simulink model "updated_target_driver_2026_withVariants_MPC_andwlqp2"  (R2024b)
settings: Solver=FixedStepDiscrete  StartTime=0.0  StopTime=running_time  FixedStep=dt_s  RelTol=1e-3
values from neighbouring files (symbols this model uses):
  A = gamma_2*gamma_3*Thrust_desired    [force2voltage.m]
  a2_lb = -0.25    [target_driver_setup_2022_Ctrl_V_2_4.m]    (also in target_driver_setup_2022_Ctrl_V_2_4_geometric.m; target_driver_setup_mpc_12msdelay.m; target_driver_setup_mpc_andWLQP.m)
  a2_openloop = -0    (= 0)    [target_driver_setup_2022_Ctrl_V_2_4.m]    (also in target_driver_setup_2022_Ctrl_V_2_4_geometric.m; target_driver_setup_mpc_12msdelay.m; target_driver_setup_mpc_andWLQP.m)
  a2_ub = 0.25    [target_driver_setup_2022_Ctrl_V_2_4.m]    (also in target_driver_setup_2022_Ctrl_V_2_4_geometric.m; target_driver_setup_mpc_12msdelay.m; target_driver_setup_mpc_andWLQP.m)
  att_s = 500    [target_driver_setup_2022_Ctrl_V_2_4.m]    (also in target_driver_setup_2022_Ctrl_V_2_4_geometric.m; target_driver_setup_mpc_12msdelay.m; target_driver_setup_mpc_andWLQP.m)
  c_vertical = 0.70e-3    (= 0.0007)    [target_driver_setup_mpc_andWLQP.m]
  closedloop_flag = 1    [target_driver_setup_2022_Ctrl_V_2_4.m]    (also in target_driver_setup_2022_Ctrl_V_2_4_geometric.m = 0; target_driver_setup_mpc_12msdelay.m = 0; target_driver_setup_mpc_andWLQP.m = 0)
  delay = delay-vicon_sample_cycle/2    [target_driver_setup_2022_Ctrl_V_2_4.m]    (also in target_driver_setup_2022_Ctrl_V_2_4_geometric.m; target_driver_setup_mpc_12msdelay.m; target_driver_setup_mpc_andWLQP.m)
  drv_amp = abs((vleft_p2p-vright_p2p))/2+min(vleft_p2p,vright_p2p)    [Wing_traj_to_Voltage.m]    (also in force2voltage.m; target_driver_setup_2022_Ctrl_V_2_4.m = 300; target_driver_setup_2022_Ctrl_V_2_4_geometric.m = 110; target_driver_setup_mpc_12msdelay.m = 150)
  drv_bias = max_drv_bias    (= 300)    [target_driver_setup_2022_Ctrl_V_2_4.m]    (also in target_driver_setup_2022_Ctrl_V_2_4_geometric.m = 200; target_driver_setup_mpc_12msdelay.m = 200; target_driver_setup_mpc_andWLQP.m = 200)
  drv_pitch_left = vleft_pitch    [Wing_traj_to_Voltage.m]    (also in force2voltage.m = 0; target_driver_setup_2022_Ctrl_V_2_4.m = 0; target_driver_setup_2022_Ctrl_V_2_4_geometric.m = 9.05; target_driver_setup_mpc_12msdelay.m = 9.05)
  drv_pitch_right = vright_pitch    [Wing_traj_to_Voltage.m]    (also in force2voltage.m = 0; target_driver_setup_2022_Ctrl_V_2_4.m = 0; target_driver_setup_2022_Ctrl_V_2_4_geometric.m = 9.05; target_driver_setup_mpc_12msdelay.m = 9.05)
  drv_roll = (vleft_p2p-vright_p2p)/4    [Wing_traj_to_Voltage.m]    (also in force2voltage.m; target_driver_setup_2022_Ctrl_V_2_4.m = 0; target_driver_setup_2022_Ctrl_V_2_4_geometric.m = -0.001; target_driver_setup_mpc_12msdelay.m = -0.001)
  dt_s = 1e-3    (= 0.001)    [target_driver_setup_2022_Ctrl_V_2_4.m]    (also in target_driver_setup_2022_Ctrl_V_2_4_geometric.m = 0.0002; target_driver_setup_mpc_12msdelay.m = 0.0002; target_driver_setup_mpc_andWLQP.m = 2.0e-4;1)
  f_fin = f    (= 180)    [target_driver_setup_2022_Ctrl_V_2_4.m]    (also in target_driver_setup_2022_Ctrl_V_2_4_geometric.m = 155; target_driver_setup_mpc_12msdelay.m = 155; target_driver_setup_mpc_andWLQP.m = 155)
  f_int = f    (= 180)    [target_driver_setup_2022_Ctrl_V_2_4.m]    (also in target_driver_setup_2022_Ctrl_V_2_4_geometric.m = 155; target_driver_setup_mpc_12msdelay.m = 155; target_driver_setup_mpc_andWLQP.m = 155)
  g = 9.8    [target_driver_setup_2022_Ctrl_V_2_4.m]    (also in target_driver_setup_2022_Ctrl_V_2_4_geometric.m; target_driver_setup_mpc_12msdelay.m; target_driver_setup_mpc_andWLQP.m = 9.81; test_full_attitude_mpc.m = 9.81)
  I_moment = eye(3)    [target_driver_exec_2022_Ctrl_V_2_4.m]    (also in target_driver_setup_2022_Ctrl_V_2_4.m; target_driver_setup_2022_Ctrl_V_2_4_geometric.m; target_driver_setup_mpc_12msdelay.m; target_driver_setup_mpc_andWLQP.m)
  k_tau_vec = [k_tau_roll;k_tau_pitch]    [target_driver_setup_2022_Ctrl_V_2_4_geometric.m]    (also in target_driver_setup_mpc_12msdelay.m; target_driver_setup_mpc_andWLQP.m)
  m = t <= t_zoom    [plot_roll_torque_cmd_vs_actual.m]    (also in plot_roll_torque_cmd_vs_actual_flightlog.m = t >= t0 & t <= t1; target_driver_setup_2022_Ctrl_V_2_4.m = 0.000124; target_driver_setup_2022_Ctrl_V_2_4_geometric.m = 8.5655e-05; target_driver_setup_mpc_12msdelay.m = 8.5655e-05)
  params_vec = [params_opt.delta_1, params_opt.delta_2, params_opt.delta_3,      params_opt.gamma_1, params_opt.gamma_2_1, params_opt.gamma_3,      params_opt.eta, params_opt.nu, params_opt.mu]'    [force2voltage_tuningSandbox.m]    (also in target_driver_setup_2022_Ctrl_V_2_4.m = [params_opt.delta_1, params_opt.delta_2, params_opt.delta_3,; target_driver_setup_2022_Ctrl_V_2_4_geometric.m = [params_opt.delta_1, params_opt.delta_2, params_opt.delta_3,; target_driver_setup_mpc_12msdelay.m = [params_opt.delta_1, params_opt.delta_2, params_opt.delta_3,; target_driver_setup_mpc_andWLQP.m = [params_opt.delta_1, params_opt.delta_2, params_opt.delta_3,)
  phase = 0    [target_driver_setup_2022_Ctrl_V_2_4.m]    (also in target_driver_setup_2022_Ctrl_V_2_4_geometric.m; target_driver_setup_mpc_12msdelay.m; target_driver_setup_mpc_andWLQP.m)
  popts_flattened = popts.popts    [target_driver_setup_mpc_andWLQP.m]
  roll_offset_angle = 0    [target_driver_setup_2022_Ctrl_V_2_4.m]    (also in target_driver_setup_2022_Ctrl_V_2_4_geometric.m; target_driver_setup_mpc_12msdelay.m; target_driver_setup_mpc_andWLQP.m)
  running_time = start_delay+total_T    (= 9)    [target_driver_setup_2022_Ctrl_V_2_4.m]    (also in target_driver_setup_2022_Ctrl_V_2_4_geometric.m = 10; target_driver_setup_mpc_12msdelay.m = 0.5; target_driver_setup_mpc_andWLQP.m = 10)
  running_time_control = start_delay_control+total_T+0.0    (= 7.1)    [target_driver_setup_2022_Ctrl_V_2_4.m]    (also in target_driver_setup_2022_Ctrl_V_2_4_geometric.m = 10; target_driver_setup_mpc_12msdelay.m = 0.5; target_driver_setup_mpc_andWLQP.m = 10)
  sampling_f = 10000    [target_driver_setup_2022_Ctrl_V_2_4.m]    (also in target_driver_setup_2022_Ctrl_V_2_4_geometric.m = 5000; target_driver_setup_mpc_12msdelay.m = 5000; target_driver_setup_mpc_andWLQP.m = 1/dt_s)
  start_delay = 2.0    (= 2)    [target_driver_setup_2022_Ctrl_V_2_4.m]    (also in target_driver_setup_2022_Ctrl_V_2_4_geometric.m = 0; target_driver_setup_mpc_12msdelay.m = 0; target_driver_setup_mpc_andWLQP.m = 0)
  start_delay_control = start_delay + ramp_delay    (= 0.1)    [target_driver_setup_2022_Ctrl_V_2_4.m]    (also in target_driver_setup_2022_Ctrl_V_2_4_geometric.m = 0; target_driver_setup_mpc_12msdelay.m = 0; target_driver_setup_mpc_andWLQP.m = 0)
  T = 1    [target_driver_setup_2022_Ctrl_V_2_4.m]    (also in target_driver_setup_2022_Ctrl_V_2_4_geometric.m = 10; target_driver_setup_mpc_12msdelay.m = 0.5; target_driver_setup_mpc_andWLQP.m = 10; test_full_attitude_mpc.m = T0 + nu(1))
  weights_vec = [ws; wds; wpr_xy;wpr_z; wpf; wvr_xy; wvr_z ... (first row only)    [target_driver_setup_2022_Ctrl_V_2_4_geometric.m]    (also in target_driver_setup_mpc_12msdelay.m; target_driver_setup_mpc_andWLQP.m)
undefined symbols (not defined in the file or in its folder): Com1, ctrl_Ts, DiscIntNeverNeededParam, dspblkCoreblockFVToolHelper, gcbh, left_mapping, left_mapping_F_to_Phi, lp_den, lp_num, none, right_mapping, right_mapping_F_to_Phi
libraries: simulink x17, xpcseriallib x2, cstblocks x1, xpcnilib x1, xpcutilitieslib x1
(part 3 of 4)

== system updated_target_driver_2026_withVariants_MPC_andwlqp2/Variant Subsystem/Simulation/signal generator a3/Drive_Signal/AveragedOffset_filtered ==
  note: To avoid having signal "jump",
      | we want SMOOTH transitions
      | in frequency (i.e., a weighted sum
      | of current freq and freq some delta t ago)
  note: time constant 0.02sec
      | for 10kHz samping
  In1 : Inport
  Discrete Transfer Fcn : DiscreteTransferFcn  LoadFcn=dspblkCoreblockFVToolHelper(gcbh,'load');  Numerator=[0.05]  Denominator=[1 -.95]
      settings: CopyFcn=dspblkCoreblockFVToolHelper(gcbh,'copy');  DeleteFcn=dspblkCoreblockFVToolHelper(gcbh,'close');  ModelCloseFcn=dspblkCoreblockFVToolHelper(gcbh,'close');  PreSaveFcn=dspblkCoreblockFVToolHelper(gcbh,'presave');  PostSaveFcn=dspblkCoreblockFVToolHelper(gcbh,'postsave');  CloseFcn=dspblkCoreblockFVToolHelper(gcbh,'close');
  Discrete Transfer Fcn2 : DiscreteTransferFcn  LoadFcn=dspblkCoreblockFVToolHelper(gcbh,'load');  Numerator=[0.37152]  Denominator=[1 -.62848]
      settings: CopyFcn=dspblkCoreblockFVToolHelper(gcbh,'copy');  DeleteFcn=dspblkCoreblockFVToolHelper(gcbh,'close');  ModelCloseFcn=dspblkCoreblockFVToolHelper(gcbh,'close');  PreSaveFcn=dspblkCoreblockFVToolHelper(gcbh,'presave');  PostSaveFcn=dspblkCoreblockFVToolHelper(gcbh,'postsave');  CloseFcn=dspblkCoreblockFVToolHelper(gcbh,'close');
  Out1 : Outport
  wires:
  In1/1 -> Discrete Transfer Fcn2/1
  Discrete Transfer Fcn2/1 -> Out1/1

== system updated_target_driver_2026_withVariants_MPC_andwlqp2/Variant Subsystem/Simulation/signal generator a3/Drive_Signal/FlattenedSine1 ==
  freq : Inport
  phase : Inport  Port=2
  a2 : Inport  Port=3
  0.1 : Gain  Gain=0.1
  1.1 : Gain  Gain=1.1
  2f : Gain  Gain=2
  2pi : Gain  Gain=2*pi
  3f : Gain  Gain=3
  Add : Sum  Inputs=+++
  Add1 : Sum
  Amplitude Correction : Subsystem  Commented=on
  AveragedAmp_filtered : Subsystem
  Product : Product
  first harmonic : Trigonometry  OutputSignalType=real
  integrate(omega*t) : DiscreteIntegrator  SampleTime=-1  ICPrevOutput=DiscIntNeverNeededParam  ICPrevScaledInput=DiscIntNeverNeededParam
  second harmonic : Trigonometry  OutputSignalType=real
  third harmonic : Trigonometry  OutputSignalType=real
  split cycle signal : Outport
  wires:
  freq/1 -> 2pi/1
  2pi/1 -> integrate(omega*t)/1
  3f/1 -> third harmonic/1
  first harmonic/1 -> 1.1/1
  third harmonic/1 -> 0.1/1
  1.1/1 -> Add/1
  Add1/1 -> first harmonic/1, 2f/1, 3f/1
  integrate(omega*t)/1 -> Add1/1
  phase/1 -> Add1/2
  2f/1 -> second harmonic/1
  0.1/1 -> Add/2
  Product/1 -> Add/3
  second harmonic/1 -> Product/1
  Add/1 -> split cycle signal/1
  a2/1 -> AveragedAmp_filtered/1(In1)
  AveragedAmp_filtered/1(Out1) -> Product/2

== system updated_target_driver_2026_withVariants_MPC_andwlqp2/Variant Subsystem/Simulation/signal generator a3/Drive_Signal/FlattenedSine_phase ==
  f : Inport
  phase : Inport  Port=2
  0.1 : Gain  Gain=0.1
  1.1 : Gain  Gain=1.1
  2pi : Gain  Gain=2*pi
  3f : Gain  Gain=3
  Add : Sum
  Sum : Sum  Inputs=|++
  first harmonic : Trigonometry  OutputSignalType=real
  integrate(omega*t) : DiscreteIntegrator  SampleTime=-1  ICPrevOutput=DiscIntNeverNeededParam  ICPrevScaledInput=DiscIntNeverNeededParam
  pi/180 : Gain  Gain=pi/180
  third harmonic : Trigonometry  OutputSignalType=real
  split cycle signal : Outport
  wires:
  f/1 -> 2pi/1
  2pi/1 -> integrate(omega*t)/1
  3f/1 -> third harmonic/1
  first harmonic/1 -> 1.1/1
  third harmonic/1 -> 0.1/1
  1.1/1 -> Add/1
  0.1/1 -> Add/2
  Add/1 -> split cycle signal/1
  Sum/1 -> first harmonic/1, 3f/1
  pi/180/1 -> Sum/2
  integrate(omega*t)/1 -> Sum/1
  phase/1 -> pi/180/1

== system updated_target_driver_2026_withVariants_MPC_andwlqp2/Variant Subsystem/Simulation/signal generator a3/Drive_Signal/SignalForRamp_binary ==
  note: Should output 1 or -1,
      | so signal ramps UP to 1
      | or DOWN to 0.
  In1 : Inport
  Add : Sum  Inputs=+-
  Compare To Zero : simulink/Logic and Bit Operations/Compare To Zero  relop=>  OutDataTypeStr=uint8  ZeroCross=off
  Constant : Constant
  Data Type Conversion : DataTypeConversion  OutDataTypeStr=double  SaturateOnIntegerOverflow=off  RndMeth=Floor
  Gain : Gain  Gain=2
  Out1 : Outport
  wires:
  In1/1 -> Compare To Zero/1
  Compare To Zero/1 -> Data Type Conversion/1
  Gain/1 -> Add/1
  Constant/1 -> Add/2
  Add/1 -> Out1/1
  Data Type Conversion/1 -> Gain/1

== system updated_target_driver_2026_withVariants_MPC_andwlqp2/Variant Subsystem/Simulation/signal generator a3/Drive_Signal/SignalForSin_binary ==
  note: We want this to stay "high" for 1
      | second after the actual "enable"
      | is turned off...
  In1 : Inport
  Compare To Zero : simulink/Logic and Bit Operations/Compare To Zero  relop=>  OutDataTypeStr=uint8  ZeroCross=off
  Data Type Conversion : DataTypeConversion  OutDataTypeStr=double  SaturateOnIntegerOverflow=off  RndMeth=Floor
  Out1 : Outport
  wires:
  In1/1 -> Compare To Zero/1
  Compare To Zero/1 -> Data Type Conversion/1
  Data Type Conversion/1 -> Out1/1

== system updated_target_driver_2026_withVariants_MPC_andwlqp2/Variant Subsystem/Simulation/signal generator a3/Drive_Signal/Sinewave ==
  In2 : Inport
  2pi : Gain  Gain=2*pi
  first harmonic : Trigonometry  OutputSignalType=real
  integrate(omega*t) : DiscreteIntegrator  SampleTime=-1  ICPrevOutput=DiscIntNeverNeededParam  ICPrevScaledInput=DiscIntNeverNeededParam
  split cycle signal : Outport
  wires:
  In2/1 -> 2pi/1
  2pi/1 -> integrate(omega*t)/1
  integrate(omega*t)/1 -> first harmonic/1
  first harmonic/1 -> split cycle signal/1

== system updated_target_driver_2026_withVariants_MPC_andwlqp2/Variant Subsystem/Simulation/signal generator a3/Drive_Signal1/AveragedAmp_filtered ==
  note: To avoid having signal "jump",
      | we want SMOOTH transitions
      | in frequency (i.e., a weighted sum
      | of current freq and freq some delta t ago)
  note: time constant 0.002sec
      | for 10kHz samping
  In1 : Inport
  Discrete Transfer Fcn1 : DiscreteTransferFcn  LoadFcn=dspblkCoreblockFVToolHelper(gcbh,'load');  Numerator=[0.05]  Denominator=[1 -.95]
      settings: CopyFcn=dspblkCoreblockFVToolHelper(gcbh,'copy');  DeleteFcn=dspblkCoreblockFVToolHelper(gcbh,'close');  ModelCloseFcn=dspblkCoreblockFVToolHelper(gcbh,'close');  PreSaveFcn=dspblkCoreblockFVToolHelper(gcbh,'presave');  PostSaveFcn=dspblkCoreblockFVToolHelper(gcbh,'postsave');  CloseFcn=dspblkCoreblockFVToolHelper(gcbh,'close');
  Discrete Transfer Fcn2 : DiscreteTransferFcn  LoadFcn=dspblkCoreblockFVToolHelper(gcbh,'load');  Numerator=[0.37152]  Denominator=[1 -.62848]
      settings: CopyFcn=dspblkCoreblockFVToolHelper(gcbh,'copy');  DeleteFcn=dspblkCoreblockFVToolHelper(gcbh,'close');  ModelCloseFcn=dspblkCoreblockFVToolHelper(gcbh,'close');  PreSaveFcn=dspblkCoreblockFVToolHelper(gcbh,'presave');  PostSaveFcn=dspblkCoreblockFVToolHelper(gcbh,'postsave');  CloseFcn=dspblkCoreblockFVToolHelper(gcbh,'close');
  Out1 : Outport
  wires:
  In1/1 -> Discrete Transfer Fcn2/1
  Discrete Transfer Fcn2/1 -> Out1/1

== system updated_target_driver_2026_withVariants_MPC_andwlqp2/Variant Subsystem/Simulation/signal generator a3/Drive_Signal1/AveragedOffset_filtered ==
  note: To avoid having signal "jump",
      | we want SMOOTH transitions
      | in frequency (i.e., a weighted sum
      | of current freq and freq some delta t ago)
  note: c
  note: time constant 0.02sec
      | for 10kHz samping
  In1 : Inport
  Discrete Transfer Fcn1 : DiscreteTransferFcn  LoadFcn=dspblkCoreblockFVToolHelper(gcbh,'load');  Numerator=[0.05]  Denominator=[1 -.95]
      settings: CopyFcn=dspblkCoreblockFVToolHelper(gcbh,'copy');  DeleteFcn=dspblkCoreblockFVToolHelper(gcbh,'close');  ModelCloseFcn=dspblkCoreblockFVToolHelper(gcbh,'close');  PreSaveFcn=dspblkCoreblockFVToolHelper(gcbh,'presave');  PostSaveFcn=dspblkCoreblockFVToolHelper(gcbh,'postsave');  CloseFcn=dspblkCoreblockFVToolHelper(gcbh,'close');
  Discrete Transfer Fcn2 : DiscreteTransferFcn  LoadFcn=dspblkCoreblockFVToolHelper(gcbh,'load');  Numerator=[0.37152]  Denominator=[1 -.62848]
      settings: CopyFcn=dspblkCoreblockFVToolHelper(gcbh,'copy');  DeleteFcn=dspblkCoreblockFVToolHelper(gcbh,'close');  ModelCloseFcn=dspblkCoreblockFVToolHelper(gcbh,'close');  PreSaveFcn=dspblkCoreblockFVToolHelper(gcbh,'presave');  PostSaveFcn=dspblkCoreblockFVToolHelper(gcbh,'postsave');  CloseFcn=dspblkCoreblockFVToolHelper(gcbh,'close');
  Out1 : Outport
  wires:
  In1/1 -> Discrete Transfer Fcn2/1
  Discrete Transfer Fcn2/1 -> Out1/1

== system updated_target_driver_2026_withVariants_MPC_andwlqp2/Variant Subsystem/Simulation/signal generator a3/Drive_Signal1/FlattenedSine1 ==
  freq : Inport
  a2 : Inport  Port=2
  0.1 : Gain  Gain=0.1
  1.1 : Gain  Gain=1.1
  2f : Gain  Gain=2
  2pi : Gain  Gain=2*pi
  3f : Gain  Gain=3
  Add : Sum  Inputs=+++
  Amplitude Correction : Subsystem  Commented=on
  AveragedAmp_filtered : Subsystem
  Product : Product
  first harmonic : Trigonometry  OutputSignalType=real
  flip : Gain  Gain=-1
  integrate(omega*t) : DiscreteIntegrator  SampleTime=-1  ICPrevOutput=DiscIntNeverNeededParam  ICPrevScaledInput=DiscIntNeverNeededParam
  second harmonic : Trigonometry  OutputSignalType=real
  third harmonic : Trigonometry  OutputSignalType=real
  split cycle signal : Outport
  wires:
  freq/1 -> 2pi/1
  2pi/1 -> integrate(omega*t)/1
  3f/1 -> third harmonic/1
  first harmonic/1 -> 1.1/1
  third harmonic/1 -> 0.1/1
  1.1/1 -> Add/1
  integrate(omega*t)/1 -> first harmonic/1, 2f/1, 3f/1
  2f/1 -> second harmonic/1
  0.1/1 -> Add/2
  Product/1 -> Add/3
  second harmonic/1 -> Product/1
  flip/1 -> Product/2
  Add/1 -> split cycle signal/1
  a2/1 -> AveragedAmp_filtered/1(In1)
  AveragedAmp_filtered/1(Out1) -> flip/1

== system updated_target_driver_2026_withVariants_MPC_andwlqp2/Variant Subsystem/Simulation/signal generator a3/Drive_Signal1/SignalForRamp_binary ==
  note: Should output 1 or -1,
      | so signal ramps UP to 1
      | or DOWN to 0.
  In1 : Inport
  Add : Sum  Inputs=+-
  Compare To Zero : simulink/Logic and Bit Operations/Compare To Zero  relop=>  OutDataTypeStr=uint8  ZeroCross=off
  Constant : Constant
  Data Type Conversion : DataTypeConversion  OutDataTypeStr=double  SaturateOnIntegerOverflow=off  RndMeth=Floor
  Gain : Gain  Gain=2
  Out1 : Outport
  wires:
  In1/1 -> Compare To Zero/1
  Compare To Zero/1 -> Data Type Conversion/1
  Gain/1 -> Add/1
  Constant/1 -> Add/2
  Add/1 -> Out1/1
  Data Type Conversion/1 -> Gain/1

== system updated_target_driver_2026_withVariants_MPC_andwlqp2/Variant Subsystem/Simulation/signal generator a3/Drive_Signal1/SignalForSin_binary ==
  note: We want this to stay "high" for 1
      | second after the actual "enable"
      | is turned off...
  In1 : Inport
  Compare To Zero : simulink/Logic and Bit Operations/Compare To Zero  relop=>  OutDataTypeStr=uint8  ZeroCross=off
  Data Type Conversion : DataTypeConversion  OutDataTypeStr=double  SaturateOnIntegerOverflow=off  RndMeth=Floor
  Out1 : Outport
  wires:
  In1/1 -> Compare To Zero/1
  Compare To Zero/1 -> Data Type Conversion/1
  Data Type Conversion/1 -> Out1/1

== system updated_target_driver_2026_withVariants_MPC_andwlqp2/Variant Subsystem/Simulation/signal generator a3/Drive_Signal1/Sine Wave ==
  In2 : Inport
  2pi : Gain  Gain=2*pi
  first harmonic : Trigonometry  OutputSignalType=real
  integrate(omega*t) : DiscreteIntegrator  SampleTime=-1  ICPrevOutput=DiscIntNeverNeededParam  ICPrevScaledInput=DiscIntNeverNeededParam
  split cycle signal : Outport
  wires:
  In2/1 -> 2pi/1
  2pi/1 -> integrate(omega*t)/1
  integrate(omega*t)/1 -> first harmonic/1
  first harmonic/1 -> split cycle signal/1

== system updated_target_driver_2026_withVariants_MPC_andwlqp2/Variant Subsystem/Experimental/signal generator a3/Drive_Signal/FlattenedSine1/Amplitude Correction ==
  y : Inport
  a2 : Inport  Port=2
  Abs : Abs  SaturateOnIntegerOverflow=off
  Constant : Constant  Value=1.2
  Constant1 : Constant  Value=1.1
  Divide : Product  Inputs=*/
  Product1 : Product
  Sqrt : Sqrt
  Subtract : Sum  Inputs=+-
  y_new : Outport
  wires:
  Constant/1 -> Subtract/1
  Subtract/1 -> Sqrt/1
  Abs/1 -> Subtract/2
  a2/1 -> Abs/1
  y/1 -> Product1/1
  Product1/1 -> y_new/1
  Divide/1 -> Product1/2
  Constant1/1 -> Divide/2
  Sqrt/1 -> Divide/1

== system updated_target_driver_2026_withVariants_MPC_andwlqp2/Variant Subsystem/Experimental/signal generator a3/Drive_Signal/FlattenedSine1/AveragedAmp_filtered ==
  note: To avoid having signal "jump",
      | we want SMOOTH transitions
      | in frequency (i.e., a weighted sum
      | of current freq and freq some delta t ago)
  note: time constant 0.002sec
      | for 10kHz samping
  In1 : Inport
  Discrete Transfer Fcn : DiscreteTransferFcn  Numerator=[0.05]  Denominator=[1 -.95]
  Out1 : Outport
  wires:
  In1/1 -> Discrete Transfer Fcn/1
  Discrete Transfer Fcn/1 -> Out1/1

== system updated_target_driver_2026_withVariants_MPC_andwlqp2/Variant Subsystem/Experimental/signal generator a3/Drive_Signal1/FlattenedSine1/Amplitude Correction ==
  y : Inport
  a2 : Inport  Port=2
  Abs : Abs  SaturateOnIntegerOverflow=off
  Constant : Constant  Value=1.2
  Constant1 : Constant  Value=1.1
  Divide : Product  Inputs=*/
  Product1 : Product
  Sqrt : Sqrt
  Subtract : Sum  Inputs=+-
  y_new : Outport
  wires:
  Constant/1 -> Subtract/1
  Subtract/1 -> Sqrt/1
  Abs/1 -> Subtract/2
  a2/1 -> Abs/1
  y/1 -> Product1/1
  Product1/1 -> y_new/1
  Divide/1 -> Product1/2
  Constant1/1 -> Divide/2
  Sqrt/1 -> Divide/1

== system updated_target_driver_2026_withVariants_MPC_andwlqp2/Variant Subsystem/Experimental/signal generator a3/Drive_Signal1/FlattenedSine1/AveragedAmp_filtered ==
  note: To avoid having signal "jump",
      | we want SMOOTH transitions
      | in frequency (i.e., a weighted sum
      | of current freq and freq some delta t ago)
  note: time constant 0.002sec
      | for 10kHz samping
  In1 : Inport
  Discrete Transfer Fcn : DiscreteTransferFcn  Numerator=[0.05]  Denominator=[1 -.95]
  Out1 : Outport
  wires:
  In1/1 -> Discrete Transfer Fcn/1
  Discrete Transfer Fcn/1 -> Out1/1

== system updated_target_driver_2026_withVariants_MPC_andwlqp2/Variant Subsystem/Simulation/signal generator a3/Drive_Signal/FlattenedSine1/Amplitude Correction ==
  y : Inport
  a2 : Inport  Port=2
  Abs : Abs  SaturateOnIntegerOverflow=off
  Constant : Constant  Value=1.2
  Constant1 : Constant  Value=1.1
  Divide : Product  Inputs=*/
  Product1 : Product
  Sqrt : Sqrt
  Subtract : Sum  Inputs=+-
  y_new : Outport
  wires:
  Constant/1 -> Subtract/1
  Subtract/1 -> Sqrt/1
  Abs/1 -> Subtract/2
  a2/1 -> Abs/1
  y/1 -> Product1/1
  Product1/1 -> y_new/1
  Divide/1 -> Product1/2
  Constant1/1 -> Divide/2
  Sqrt/1 -> Divide/1

== system updated_target_driver_2026_withVariants_MPC_andwlqp2/Variant Subsystem/Simulation/signal generator a3/Drive_Signal/FlattenedSine1/AveragedAmp_filtered ==
  note: To avoid having signal "jump",
      | we want SMOOTH transitions
      | in frequency (i.e., a weighted sum
      | of current freq and freq some delta t ago)
  note: time constant 0.002sec
      | for 10kHz samping
  In1 : Inport
  Discrete Transfer Fcn : DiscreteTransferFcn  Numerator=[0.05]  Denominator=[1 -.95]
  Out1 : Outport
  wires:
  In1/1 -> Discrete Transfer Fcn/1
  Discrete Transfer Fcn/1 -> Out1/1

== system updated_target_driver_2026_withVariants_MPC_andwlqp2/Variant Subsystem/Simulation/signal generator a3/Drive_Signal1/FlattenedSine1/Amplitude Correction ==
  y : Inport
  a2 : Inport  Port=2
  Abs : Abs  SaturateOnIntegerOverflow=off
  Constant : Constant  Value=1.2
  Constant1 : Constant  Value=1.1
  Divide : Product  Inputs=*/
  Product1 : Product
  Sqrt : Sqrt
  Subtract : Sum  Inputs=+-
  y_new : Outport
  wires:
  Constant/1 -> Subtract/1
  Subtract/1 -> Sqrt/1
  Abs/1 -> Subtract/2
  a2/1 -> Abs/1
  y/1 -> Product1/1
  Product1/1 -> y_new/1
  Divide/1 -> Product1/2
  Constant1/1 -> Divide/2
  Sqrt/1 -> Divide/1

== system updated_target_driver_2026_withVariants_MPC_andwlqp2/Variant Subsystem/Simulation/signal generator a3/Drive_Signal1/FlattenedSine1/AveragedAmp_filtered ==
  note: To avoid having signal "jump",
      | we want SMOOTH transitions
      | in frequency (i.e., a weighted sum
      | of current freq and freq some delta t ago)
  note: time constant 0.002sec
      | for 10kHz samping
  In1 : Inport
  Discrete Transfer Fcn : DiscreteTransferFcn  Numerator=[0.05]  Denominator=[1 -.95]
  Out1 : Outport
  wires:
  In1/1 -> Discrete Transfer Fcn/1
  Discrete Transfer Fcn/1 -> Out1/1

== matlab function updated_target_driver_2026_withVariants_MPC_andwlqp2/Variant Subsystem/Simulation/Drake 2 Controller Axes1 ==
  data: x_drake input; x output; y_drake input; z_drake input; y output; z output
function [x,y,z] = fcn(x_drake,y_drake,z_drake)

    [x,y,z] = drake2controllerposition(x_drake,y_drake,z_drake); 

end

== matlab function updated_target_driver_2026_withVariants_MPC_andwlqp2/MATLAB Function1 ==
  data: R_cur input size=9; pdotdes output size=6; omega input size=3; p_cur input size=3; v_cur input size=3; pdes input size=3; dpdes input size=3; sdes_in input size=3; I_moment_vec input size=3; m input size=1; g input size=1; cntrl_enable input size=1; weights_vec input size=14; k_tau input size=2; ctrl_Ts input size=1; h0_wl output size=6; accdes output size=6; thrust_desired output size=1; roll_torque_desired output size=1; pitch_torque_desired output size=1; yaw_torque_desired output size=1; a_ref input; yaw_ref input
function [pdotdes, h0_wl, accdes, thrust_desired, roll_torque_desired, ...
    pitch_torque_desired, yaw_torque_desired] = fcn( ...
    R_cur, omega, p_cur, v_cur, pdes, dpdes, sdes_in, ...
    I_moment_vec, m, g, cntrl_enable, weights_vec, k_tau, ctrl_Ts, a_ref, yaw_ref) 

%#codegen
    [pdotdes, h0_wl, accdes, thrust_desired, roll_torque_desired, ...
    pitch_torque_desired, yaw_torque_desired] = upright_template_mpc_wl( ...
    R_cur, omega, p_cur, v_cur, pdes, dpdes, sdes_in, ...
    I_moment_vec, m, g, cntrl_enable, weights_vec, k_tau, ctrl_Ts, a_ref, yaw_ref); 

end

== matlab function updated_target_driver_2026_withVariants_MPC_andwlqp2/wlqp2driver ==
  data: u input size=4; drv_amp output size=1; drv_pitch_left output size=1; drv_pitch_right output size=1; drv_roll output size=1; a2 output size=1; signs input size=3; drv_bias output size=1; vleft output size=1; vright output size=1
function [drv_amp, drv_pitch_left, drv_pitch_right, drv_roll, a2, ...
    drv_bias, vleft, vright] = fcn(u, signs)
    [drv_amp, drv_pitch_left, drv_pitch_right, drv_roll, a2, ...
    drv_bias, vleft, vright] = wlqp2driver(u, signs);
end

== matlab function updated_target_driver_2026_withVariants_MPC_andwlqp2/Force to voltage/Control Mode/Force_to_Voltage1/Desired_Force_to_Voltage ==
  data: Thrust_desired input; drv_amp output; Roll_torque_desired input; Pitch_torque_desired input; Yaw_torque_desired input; drv_roll output; drv_pitch_left output; drv_pitch_right output; a2_coeff output; params_vec input
function [drv_amp, drv_roll, drv_pitch_left, drv_pitch_right, a2_coeff] =    fcn(Thrust_desired, Roll_torque_desired, Pitch_torque_desired, Yaw_torque_desired, params_vec)

% 
% Thrust_desired = 0.7e-3;% N
% Roll_torque_desired = 20e-6; %mN mm 
% Pitch_torque_desired = 0;% N  
% Yaw_torque_desired = 0;  
[drv_amp, drv_roll, drv_pitch_left, drv_pitch_right, a2_coeff] = force2voltage( ...
    Thrust_desired, Roll_torque_desired, Pitch_torque_desired, ...
    Yaw_torque_desired, params_vec);
% % global params_opt
% 
% delta_1 = params_vec(1);
% delta_2 = params_vec(2);
% delta_3 = params_vec(3);
% gamma_1 = params_vec(4);
% gamma_2 = params_vec(5);
% gamma_3 = params_vec(6);
% eta = params_vec(7);
% nu = params_vec(8);
% mu = params_vec(9);
% 
% 
% % Initializing for averaging filter at the end to prevent InF
% if Thrust_desired==0    
%     u4 = 0;
% else
%     u4 = Pitch_torque_desired/(Thrust_desired*delta_3*gamma_2)-nu;
% end
% 
% 
% % u3 calculation when tau approaches to zero
% if abs(Yaw_torque_desired)<1e-12
% 
%    u3 = -mu;
% else
%     % Bounds for the mapping to produce real solution
%     lb =(Thrust_desired/2)*(gamma_2*gamma_3*delta_2*mu/delta_1-sqrt((gamma_2*gamma_3*delta_2*Thrust_desired*mu/delta_1)^2+gamma_2*gamma_3));
%     ub =(Thrust_desired/2)*(gamma_2*gamma_3*delta_2*mu/delta_1+sqrt((gamma_2*gamma_3*delta_2*Thrust_desired*mu/delta_1)^2+gamma_2*gamma_3));
% 
%     if Yaw_torque_desired>=ub
%        Yaw_torque_desired = ub;
%     elseif Yaw_torque_desired<=lb
%        Yaw_torque_desired = lb; 
%     end
% 
%     % u3 calculation when tau approaches zero
%     if abs(Yaw_torque_desired) < 1e-12
%         u3 = -mu;
%     else
%         A = gamma_2*gamma_3*Thrust_desired;
%         B = gamma_2*gamma_3*delta_2*Thrust_desired*mu/delta_1;
% 
%         disc = A^2 - 4*Yaw_torque_desired*(Yaw_torque_desired - B);
% 
%     % Numerical / feasibility guard
%     if disc < 0
%         disc = 0;
%     end
% 
%     u3 = delta_1*(A - sqrt(disc))/(2*delta_2*Yaw_torque_desired);
%     end
% end
% 
% D = delta_1^2+delta_2^2*u3^2;
% % gamma_2*Thrust_desired+Roll_torque_desired 
% u1 = (gamma_2*Thrust_desired+Roll_torque_desired)/(2*gamma_1*gamma_2*D*eta);
% u2 = (gamma_2*Thrust_desired-Roll_torque_desired)/(2*gamma_1*gamma_2*D);
% 
% u1 = max(u1, 0); 
% u2 = max(u2, 0); % Guard against negative voltage
% vleft_p2p = sqrt(u1)*2; 
% vright_p2p = sqrt(u2)*2;
% vleft_pitch = u4;
% vright_pitch = u4;
% 
% 
% drv_amp = abs((vleft_p2p-vright_p2p))/2+min(vleft_p2p,vright_p2p); % p2p
% drv_roll = (vleft_p2p-vright_p2p)/4; % Amplitude
% drv_pitch_left = vleft_pitch;
% drv_pitch_right = vright_pitch;
% a2_coeff = u3;
% 
end

== matlab function updated_target_driver_2026_withVariants_MPC_andwlqp2/MATLAB Function2 ==
  data: Rot_corrected_vec input; wrenchBias output; v_filtered_W input; c_vertical_N_per_mps input
function wrenchBias = wlqp_vertical_wrench_bias(Rot_corrected_vec, v_filtered_W, c_vertical_N_per_mps)
%#codegen
    wrenchBias = wlqp_vertical_wrench_bias( ...
    Rot_corrected_vec, v_filtered_W, c_vertical_N_per_mps); 
end 

% y = u;

== matlab function updated_target_driver_2026_withVariants_MPC_andwlqp2/Force to voltage/Control Mode/Force_to_Voltage1/Force to Trajectory  ==
  data: Thrust_desired input; Phi_left_p2p_desired output; Roll_torque_desired input; Pitch_torque_desired input; left_mapping_F_to_Phi input; right_mapping_F_to_Phi input; A input; Phi_right_p2p_desired output; Phi_pitch_desired output
function [Phi_left_p2p_desired, Phi_right_p2p_desired, Phi_pitch_desired] = fcn(Thrust_desired, Roll_torque_desired, Pitch_torque_desired, left_mapping_F_to_Phi, right_mapping_F_to_Phi, A)

delta_opt_L = left_mapping_F_to_Phi(1);
gamma_opt_L = left_mapping_F_to_Phi(2);
phi_opt_L = left_mapping_F_to_Phi(3);
phi_opt_offset_L = left_mapping_F_to_Phi(4);

delta_opt_R = right_mapping_F_to_Phi(1);
gamma_opt_R = right_mapping_F_to_Phi(2);
phi_opt_R = right_mapping_F_to_Phi(3);
phi_opt_offset_R = right_mapping_F_to_Phi(4);

T_thrust_roll = A*[ delta_opt_L              ,               delta_opt_R;...
                    delta_opt_L*gamma_opt_L  , - delta_opt_R*gamma_opt_R];
T_pitch_thrust = A*[delta_opt_L*gamma_opt_L  , delta_opt_R*gamma_opt_R].*[phi_opt_L, phi_opt_R];
T_pitch_offset = A*[delta_opt_L*gamma_opt_L  , delta_opt_R*gamma_opt_R].*[phi_opt_offset_L, phi_opt_offset_R];

Thrust_roll = [Thrust_desired; Roll_torque_desired];
u1_u2_desired = (T_thrust_roll)\Thrust_roll;

if (T_pitch_thrust*u1_u2_desired)==0
	Phi_pitch_desired = 0;
else
	Phi_pitch_desired = (Pitch_torque_desired-T_pitch_offset*u1_u2_desired)/(T_pitch_thrust*u1_u2_desired);
end

Phi_left_p2p_desired = sqrt(u1_u2_desired(1));
Phi_right_p2p_desired = sqrt(u1_u2_desired(2));

== matlab function updated_target_driver_2026_withVariants_MPC_andwlqp2/Force to voltage/Control Mode/Force_to_Voltage1/Trajectory to Voltage Input  ==
  data: Phi_left_p2p_command input; drv_amp output; Phi_right_p2p_command input; Phi_pitch_command input; drv_roll output; drv_pitch_left output; left_mapping input; right_mapping input; drv_pitch_right output
function [drv_amp, drv_roll, drv_pitch_left, drv_pitch_right] = fcn(Phi_left_p2p_command,Phi_right_p2p_command,Phi_pitch_command,left_mapping,right_mapping)

% Mapping for Voltage peak to peak from desired Stroke peak to peak
p1_left = left_mapping(1); % V_left_p2p = p1_left*Phi_p2p + p2_left
p2_left = left_mapping(2);
p1_right = right_mapping(1); % V_right_p2p = p1_right*Phi_p2p + p2_right
p2_right = right_mapping(2);

% Mapping for Voltage offset to peak from desired Stroke peak to peak
p1_pitch_left = left_mapping(3); % vleft_pitch = p1_pitch_left*Phi_pitch_command + p2_pitch_left
p2_pitch_left = left_mapping(4);
p1_pitch_right = right_mapping(3); % vright_pitch = p1_pitch_right*Phi_pitch_command + p2_pitch_right
p2_pitch_right = right_mapping(4);

vleft_p2p = p1_left*Phi_left_p2p_command + p2_left;
vright_p2p = p1_right*Phi_right_p2p_command + p2_right;
vleft_pitch = p1_pitch_left*Phi_pitch_command + p2_pitch_left;
vright_pitch = p1_pitch_right*Phi_pitch_command + p2_pitch_right;



drv_amp = abs((vleft_p2p-vright_p2p))/2+min(vleft_p2p,vright_p2p); % p2p
drv_roll = (vleft_p2p-vright_p2p)/4; % Amplitude
drv_pitch_left = vleft_pitch;
drv_pitch_right = vright_pitch;

== matlab function updated_target_driver_2026_withVariants_MPC_andwlqp2/Force to voltage/Replay Mode/Force_to_Voltage1/Desired_Force_to_Voltage ==
  data: Thrust_desired input; drv_amp output; Roll_torque_desired input; Pitch_torque_desired input; Yaw_torque_desired input; drv_roll output; drv_pitch_left output; drv_pitch_right output; a2_coeff output; params_vec input
function [drv_amp, drv_roll, drv_pitch_left, drv_pitch_right, a2_coeff] =    fcn(Thrust_desired, Roll_torque_desired, Pitch_torque_desired, Yaw_torque_desired, params_vec)

% 
% Thrust_desired = 0.7e-3;% N
% Roll_torque_desired = 20e-6; %mN mm 
% Pitch_torque_desired = 0;% N  
% Yaw_torque_desired = 0;  
[drv_amp, drv_roll, drv_pitch_left, drv_pitch_right, a2_coeff] = force2voltage( ...
    Thrust_desired, Roll_torque_desired, Pitch_torque_desired, ...
    Yaw_torque_desired, params_vec);
% % global params_opt
% 
% delta_1 = params_vec(1);
% delta_2 = params_vec(2);
% delta_3 = params_vec(3);
% gamma_1 = params_vec(4);
% gamma_2 = params_vec(5);
% gamma_3 = params_vec(6);
% eta = params_vec(7);
% nu = params_vec(8);
% mu = params_vec(9);
% 
% 
% % Initializing for averaging filter at the end to prevent InF
% if Thrust_desired==0    
%     u4 = 0;
% else
%     u4 = Pitch_torque_desired/(Thrust_desired*delta_3*gamma_2)-nu;
% end
% 
% 
% % u3 calculation when tau approaches to zero
% if abs(Yaw_torque_desired)<1e-12
% 
%    u3 = -mu;
% else
%     % Bounds for the mapping to produce real solution
%     lb =(Thrust_desired/2)*(gamma_2*gamma_3*delta_2*mu/delta_1-sqrt((gamma_2*gamma_3*delta_2*Thrust_desired*mu/delta_1)^2+gamma_2*gamma_3));
%     ub =(Thrust_desired/2)*(gamma_2*gamma_3*delta_2*mu/delta_1+sqrt((gamma_2*gamma_3*delta_2*Thrust_desired*mu/delta_1)^2+gamma_2*gamma_3));
% 
%     if Yaw_torque_desired>=ub
%        Yaw_torque_desired = ub;
%     elseif Yaw_torque_desired<=lb
%        Yaw_torque_desired = lb; 
%     end
% 
%     % u3 calculation when tau approaches zero
%     if abs(Yaw_torque_desired) < 1e-12
%         u3 = -mu;
%     else
%         A = gamma_2*gamma_3*Thrust_desired;
%         B = gamma_2*gamma_3*delta_2*Thrust_desired*mu/delta_1;
% 
%         disc = A^2 - 4*Yaw_torque_desired*(Yaw_torque_desired - B);
% 
%     % Numerical / feasibility guard
%     if disc < 0
%         disc = 0;
%     end
% 
%     u3 = delta_1*(A - sqrt(disc))/(2*delta_2*Yaw_torque_desired);
%     end
% end
% 
% D = delta_1^2+delta_2^2*u3^2;
% % gamma_2*Thrust_desired+Roll_torque_desired 
% u1 = (gamma_2*Thrust_desired+Roll_torque_desired)/(2*gamma_1*gamma_2*D*eta);
% u2 = (gamma_2*Thrust_desired-Roll_torque_desired)/(2*gamma_1*gamma_2*D);
% 
% u1 = max(u1, 0); 
% u2 = max(u2, 0); % Guard against negative voltage
% vleft_p2p = sqrt(u1)*2; 
% vright_p2p = sqrt(u2)*2;
% vleft_pitch = u4;
% vright_pitch = u4;
% 
% 
% drv_amp = abs((vleft_p2p-vright_p2p))/2+min(vleft_p2p,vright_p2p); % p2p
% drv_roll = (vleft_p2p-vright_p2p)/4; % Amplitude
% drv_pitch_left = vleft_pitch;
% drv_pitch_right = vright_pitch;
% a2_coeff = u3;
% 
end

== matlab function updated_target_driver_2026_withVariants_MPC_andwlqp2/Force to voltage/Replay Mode/Force_to_Voltage1/Force to Trajectory  ==
  data: Thrust_desired input; Phi_left_p2p_desired output; Roll_torque_desired input; Pitch_torque_desired input; left_mapping_F_to_Phi input; right_mapping_F_to_Phi input; A input; Phi_right_p2p_desired output; Phi_pitch_desired output
function [Phi_left_p2p_desired, Phi_right_p2p_desired, Phi_pitch_desired] = fcn(Thrust_desired, Roll_torque_desired, Pitch_torque_desired, left_mapping_F_to_Phi, right_mapping_F_to_Phi, A)

delta_opt_L = left_mapping_F_to_Phi(1);
gamma_opt_L = left_mapping_F_to_Phi(2);
phi_opt_L = left_mapping_F_to_Phi(3);
phi_opt_offset_L = left_mapping_F_to_Phi(4);

delta_opt_R = right_mapping_F_to_Phi(1);
gamma_opt_R = right_mapping_F_to_Phi(2);
phi_opt_R = right_mapping_F_to_Phi(3);
phi_opt_offset_R = right_mapping_F_to_Phi(4);

T_thrust_roll = A*[ delta_opt_L              ,               delta_opt_R;...
                    delta_opt_L*gamma_opt_L  , - delta_opt_R*gamma_opt_R];
T_pitch_thrust = A*[delta_opt_L*gamma_opt_L  , delta_opt_R*gamma_opt_R].*[phi_opt_L, phi_opt_R];
T_pitch_offset = A*[delta_opt_L*gamma_opt_L  , delta_opt_R*gamma_opt_R].*[phi_opt_offset_L, phi_opt_offset_R];

Thrust_roll = [Thrust_desired; Roll_torque_desired];
u1_u2_desired = (T_thrust_roll)\Thrust_roll;

if (T_pitch_thrust*u1_u2_desired)==0
	Phi_pitch_desired = 0;
else
	Phi_pitch_desired = (Pitch_torque_desired-T_pitch_offset*u1_u2_desired)/(T_pitch_thrust*u1_u2_desired);
end

Phi_left_p2p_desired = sqrt(u1_u2_desired(1));
Phi_right_p2p_desired = sqrt(u1_u2_desired(2));

== matlab function updated_target_driver_2026_withVariants_MPC_andwlqp2/Force to voltage/Replay Mode/Force_to_Voltage1/Trajectory to Voltage Input  ==
  data: Phi_left_p2p_command input; drv_amp output; Phi_right_p2p_command input; Phi_pitch_command input; drv_roll output; drv_pitch_left output; left_mapping input; right_mapping input; drv_pitch_right output
function [drv_amp, drv_roll, drv_pitch_left, drv_pitch_right] = fcn(Phi_left_p2p_command,Phi_right_p2p_command,Phi_pitch_command,left_mapping,right_mapping)

% Mapping for Voltage peak to peak from desired Stroke peak to peak
p1_left = left_mapping(1); % V_left_p2p = p1_left*Phi_p2p + p2_left
p2_left = left_mapping(2);
p1_right = right_mapping(1); % V_right_p2p = p1_right*Phi_p2p + p2_right
p2_right = right_mapping(2);

% Mapping for Voltage offset to peak from desired Stroke peak to peak
p1_pitch_left = left_mapping(3); % vleft_pitch = p1_pitch_left*Phi_pitch_command + p2_pitch_left
p2_pitch_left = left_mapping(4);
p1_pitch_right = right_mapping(3); % vright_pitch = p1_pitch_right*Phi_pitch_command + p2_pitch_right
p2_pitch_right = right_mapping(4);

vleft_p2p = p1_left*Phi_left_p2p_command + p2_left;
vright_p2p = p1_right*Phi_right_p2p_command + p2_right;
vleft_pitch = p1_pitch_left*Phi_pitch_command + p2_pitch_left;
vright_pitch = p1_pitch_right*Phi_pitch_command + p2_pitch_right;



drv_amp = abs((vleft_p2p-vright_p2p))/2+min(vleft_p2p,vright_p2p); % p2p
drv_roll = (vleft_p2p-vright_p2p)/4; % Amplitude
drv_pitch_left = vleft_pitch;
drv_pitch_right = vright_pitch;

== matlab function updated_target_driver_2026_withVariants_MPC_andwlqp2/Force_to_Voltage1/Desired_Force_to_Voltage ==
  data: Thrust_desired input; drv_amp output; Roll_torque_desired input; Pitch_torque_desired input; Yaw_torque_desired input; drv_roll output; drv_pitch_left output; drv_pitch_right output; a2_coeff output; params_vec input
function [drv_amp, drv_roll, drv_pitch_left, drv_pitch_right, a2_coeff] =    fcn(Thrust_desired, Roll_torque_desired, Pitch_torque_desired, Yaw_torque_desired, params_vec)

% 
% Thrust_desired = 0.7e-3;% N
% Roll_torque_desired = 20e-6; %mN mm 
% Pitch_torque_desired = 0;% N  
% Yaw_torque_desired = 0;  
[drv_amp, drv_roll, drv_pitch_left, drv_pitch_right, a2_coeff] = force2voltage( ...
    Thrust_desired, Roll_torque_desired, Pitch_torque_desired, ...
    Yaw_torque_desired, params_vec);
% % global params_opt
% 
% delta_1 = params_vec(1);
% delta_2 = params_vec(2);
% delta_3 = params_vec(3);
% gamma_1 = params_vec(4);
% gamma_2 = params_vec(5);
% gamma_3 = params_vec(6);
% eta = params_vec(7);
% nu = params_vec(8);
% mu = params_vec(9);
% 
% 
% % Initializing for averaging filter at the end to prevent InF
% if Thrust_desired==0    
%     u4 = 0;
% else
%     u4 = Pitch_torque_desired/(Thrust_desired*delta_3*gamma_2)-nu;
% end
% 
% 
% % u3 calculation when tau approaches to zero
% if abs(Yaw_torque_desired)<1e-12
% 
%    u3 = -mu;
% else
%     % Bounds for the mapping to produce real solution
%     lb =(Thrust_desired/2)*(gamma_2*gamma_3*delta_2*mu/delta_1-sqrt((gamma_2*gamma_3*delta_2*Thrust_desired*mu/delta_1)^2+gamma_2*gamma_3));
%     ub =(Thrust_desired/2)*(gamma_2*gamma_3*delta_2*mu/delta_1+sqrt((gamma_2*gamma_3*delta_2*Thrust_desired*mu/delta_1)^2+gamma_2*gamma_3));
% 
%     if Yaw_torque_desired>=ub
%        Yaw_torque_desired = ub;
%     elseif Yaw_torque_desired<=lb
%        Yaw_torque_desired = lb; 
%     end
% 
%     % u3 calculation when tau approaches zero
%     if abs(Yaw_torque_desired) < 1e-12
%         u3 = -mu;
%     else
%         A = gamma_2*gamma_3*Thrust_desired;
%         B = gamma_2*gamma_3*delta_2*Thrust_desired*mu/delta_1;
% 
%         disc = A^2 - 4*Yaw_torque_desired*(Yaw_torque_desired - B);
% 
%     % Numerical / feasibility guard
%     if disc < 0
%         disc = 0;
%     end
% 
%     u3 = delta_1*(A - sqrt(disc))/(2*delta_2*Yaw_torque_desired);
%     end
% end
% 
% D = delta_1^2+delta_2^2*u3^2;
% % gamma_2*Thrust_desired+Roll_torque_desired 
% u1 = (gamma_2*Thrust_desired+Roll_torque_desired)/(2*gamma_1*gamma_2*D*eta);
% u2 = (gamma_2*Thrust_desired-Roll_torque_desired)/(2*gamma_1*gamma_2*D);
% 
% u1 = max(u1, 0); 
% u2 = max(u2, 0); % Guard against negative voltage
% vleft_p2p = sqrt(u1)*2; 
% vright_p2p = sqrt(u2)*2;
% vleft_pitch = u4;
% vright_pitch = u4;
% 
% 
% drv_amp = abs((vleft_p2p-vright_p2p))/2+min(vleft_p2p,vright_p2p); % p2p
% drv_roll = (vleft_p2p-vright_p2p)/4; % Amplitude
% drv_pitch_left = vleft_pitch;
% drv_pitch_right = vright_pitch;
% a2_coeff = u3;
% 
end

== matlab function updated_target_driver_2026_withVariants_MPC_andwlqp2/Force_to_Voltage1/Force to Trajectory  ==
  data: Thrust_desired input; Phi_left_p2p_desired output; Roll_torque_desired input; Pitch_torque_desired input; left_mapping_F_to_Phi input; right_mapping_F_to_Phi input; A input; Phi_right_p2p_desired output; Phi_pitch_desired output
function [Phi_left_p2p_desired, Phi_right_p2p_desired, Phi_pitch_desired] = fcn(Thrust_desired, Roll_torque_desired, Pitch_torque_desired, left_mapping_F_to_Phi, right_mapping_F_to_Phi, A)

delta_opt_L = left_mapping_F_to_Phi(1);
gamma_opt_L = left_mapping_F_to_Phi(2);
phi_opt_L = left_mapping_F_to_Phi(3);
phi_opt_offset_L = left_mapping_F_to_Phi(4);

delta_opt_R = right_mapping_F_to_Phi(1);
gamma_opt_R = right_mapping_F_to_Phi(2);
phi_opt_R = right_mapping_F_to_Phi(3);
phi_opt_offset_R = right_mapping_F_to_Phi(4);

T_thrust_roll = A*[ delta_opt_L              ,               delta_opt_R;...
                    delta_opt_L*gamma_opt_L  , - delta_opt_R*gamma_opt_R];
T_pitch_thrust = A*[delta_opt_L*gamma_opt_L  , delta_opt_R*gamma_opt_R].*[phi_opt_L, phi_opt_R];
T_pitch_offset = A*[delta_opt_L*gamma_opt_L  , delta_opt_R*gamma_opt_R].*[phi_opt_offset_L, phi_opt_offset_R];

Thrust_roll = [Thrust_desired; Roll_torque_desired];
u1_u2_desired = (T_thrust_roll)\Thrust_roll;

if (T_pitch_thrust*u1_u2_desired)==0
	Phi_pitch_desired = 0;
else
	Phi_pitch_desired = (Pitch_torque_desired-T_pitch_offset*u1_u2_desired)/(T_pitch_thrust*u1_u2_desired);
end

Phi_left_p2p_desired = sqrt(u1_u2_desired(1));
Phi_right_p2p_desired = sqrt(u1_u2_desired(2));

== matlab function updated_target_driver_2026_withVariants_MPC_andwlqp2/Variant Subsystem/Simulation/Drake 2 Controller Axes ==
  data: alpha input; rol_c output; beta input; gamma input; pitch_c output; yaw_c output
function [rol_c,pitch_c,yaw_c] = fcn(alpha,beta,gamma)

    [rol_c,pitch_c,yaw_c] = drake2controller(alpha,beta,gamma); 

end

== matlab function updated_target_driver_2026_withVariants_MPC_andwlqp2/Force_to_Voltage1/Trajectory to Voltage Input  ==
  data: Phi_left_p2p_command input; drv_amp output; Phi_right_p2p_command input; Phi_pitch_command input; drv_roll output; drv_pitch_left output; left_mapping input; right_mapping input; drv_pitch_right output
function [drv_amp, drv_roll, drv_pitch_left, drv_pitch_right] = fcn(Phi_left_p2p_command,Phi_right_p2p_command,Phi_pitch_command,left_mapping,right_mapping)

% Mapping for Voltage peak to peak from desired Stroke peak to peak
p1_left = left_mapping(1); % V_left_p2p = p1_left*Phi_p2p + p2_left
p2_left = left_mapping(2);
p1_right = right_mapping(1); % V_right_p2p = p1_right*Phi_p2p + p2_right
p2_right = right_mapping(2);

% Mapping for Voltage offset to peak from desired Stroke peak to peak
p1_pitch_left = left_mapping(3); % vleft_pitch = p1_pitch_left*Phi_pitch_command + p2_pitch_left
p2_pitch_left = left_mapping(4);
p1_pitch_right = right_mapping(3); % vright_pitch = p1_pitch_right*Phi_pitch_command + p2_pitch_right
p2_pitch_right = right_mapping(4);

vleft_p2p = p1_left*Phi_left_p2p_command + p2_left;
vright_p2p = p1_right*Phi_right_p2p_command + p2_right;
vleft_pitch = p1_pitch_left*Phi_pitch_command + p2_pitch_left;
vright_pitch = p1_pitch_right*Phi_pitch_command + p2_pitch_right;



drv_amp = abs((vleft_p2p-vright_p2p))/2+min(vleft_p2p,vright_p2p); % p2p
drv_roll = (vleft_p2p-vright_p2p)/4; % Amplitude
drv_pitch_left = vleft_pitch;
drv_pitch_right = vright_pitch;

== matlab function updated_target_driver_2026_withVariants_MPC_andwlqp2/Observer for averaged system1/Attitude Observer/Geometric Averaging Rotation Matix/Averaged quaternion ==
  data: R input; quat output
function quat = fcn(R)
Rot = zeros(3,3);
Rot = [R(1), R(2), R(3); R(4), R(5), R(6); R(7), R(8), R(9); ];
quat = rotm2quat(Rot)';

== matlab function updated_target_driver_2026_withVariants_MPC_andwlqp2/Observer for averaged system1/Attitude Observer/Geometric Averaging Rotation Matix/Geometric Averaging Rotation M/Geometric Average  ==
  data: R_prev input; R_prev2 input; R_prev3 input; R_prev4 input; R_prev5 input; R_prev6 input; Rout output; R_cur input; update input; Rout_prev input
function Rout = fcn(R_prev,R_prev2,R_prev3,R_prev4,R_prev5,R_prev6,R_cur,update,Rout_prev)
%#codegen
% Average recent rotation matrices safely near small angles.
%
% Inputs are 9-vectors using row-major packing:
% R_vec = [R(1,1); R(1,2); R(1,3);
%          R(2,1); R(2,2); R(2,3);
%          R(3,1); R(3,2); R(3,3)]
%
% Output uses the same row-major packing.

Rout = zeros(9,1);

R_cur      = reshape(R_cur,9,1);
R_prev     = reshape(R_prev,9,1);
R_prev2    = reshape(R_prev2,9,1);
R_prev3    = reshape(R_prev3,9,1);
R_prev4    = reshape(R_prev4,9,1); %#ok<NASGU>
R_prev5    = reshape(R_prev5,9,1); %#ok<NASGU>
R_prev6    = reshape(R_prev6,9,1); %#ok<NASGU>
Rout_prev  = reshape(Rout_prev,9,1);

% Reconstruct row-major 9-vector into 3x3 matrix.
Rot_cur   = vec_to_rotm(R_cur);
Rot_prev  = vec_to_rotm(R_prev);
Rot_prev2 = vec_to_rotm(R_prev2);
Rot_prev3 = vec_to_rotm(R_prev3);

if update > 0
    Rout = Rout_prev;
else
    % 1-cycle / 4-sample average.
    %
    % IMPORTANT:
    % Do not do sign correction like w = -w here.
    % That is valid for quaternions, but not for rotation vectors.
    w_R0 = log_so3(Rot_cur);
    w_R1 = log_so3(Rot_prev);
    w_R2 = log_so3(Rot_prev2);
    w_R3 = log_so3(Rot_prev3);

    w_mean = (w_R0 + w_R1 + w_R2 + w_R3) / 4.0;

    mean_R = exp_so3(w_mean);

    % Optional but useful: project back to SO(3) to remove tiny numerical drift.
    mean_R = project_to_so3(mean_R);

    Rout = rotm_to_vec(mean_R);
end

end


function R = vec_to_rotm(R_vec)
% Convert row-major 9-vector to 3x3 matrix.

R = [R_vec(1), R_vec(2), R_vec(3);
     R_vec(4), R_vec(5), R_vec(6);
     R_vec(7), R_vec(8), R_vec(9)];
end


function R_vec = rotm_to_vec(R)
% Convert 3x3 matrix to row-major 9-vector.

R_vec = [R(1,1);
         R(1,2);
         R(1,3);
         R(2,1);
         R(2,2);
         R(2,3);
         R(3,1);
         R(3,2);
         R(3,3)];
end


function w = log_so3(R)
% Small-angle-safe logarithm map from SO(3) to rotation vector.
%
% For small theta, avoid theta/(sin(theta)) numerical issues.

c = (trace(R) - 1.0) / 2.0;

% Clamp for numerical safety.
if c > 1.0
    c = 1.0;
elseif c < -1.0
    c = -1.0;
end

theta = acos(c);

vee_part = [R(3,2) - R(2,3);
            R(1,3) - R(3,1);
            R(2,1) - R(1,2)];

if theta < 1.0e-6
    % Since R - R' ~= 2*w_hat for small rotations.
    w = 0.5 * vee_part;
else
    s = sin(theta);

    if abs(s) < 1.0e-9
        % Near pi is not expected in hover, but this avoids division blow-up.
        % Fall back to small-angle style approximation rather than producing NaN.
        w = 0.5 * vee_part;
    else
        w = theta / (2.0 * s) * vee_part;
    end
end

end


function R = exp_so3(w)
% Small-angle-safe exponential map from rotation vector to SO(3).

theta = norm(w);

W = [0.0,   -w(3),  w(2);
     w(3),   0.0,  -w(1);
    -w(2),   w(1),  0.0];

if theta < 1.0e-6
    % Rodrigues small-angle expansion.
    R = eye(3) + W + 0.5 * (W * W);
else
    R = eye(3) ...
        + (sin(theta) / theta) * W ...
        + ((1.0 - cos(theta)) / (theta * theta)) * (W * W);
end

end


function R_out = project_to_so3(R_in)
% Project a near-rotation matrix back to SO(3).
% This prevents slow drift from numerical errors.

[U,~,V] = svd(R_in);
R_out = U * V';

if det(R_out) < 0
    U(:,3) = -U(:,3);
    R_out = U * V';
end

end

== matlab function updated_target_driver_2026_withVariants_MPC_andwlqp2/Observer for averaged system1/Attitude Observer/Geometric Averaging Rotation Matix/Raw quaternion ==
  data: R input; quat output
function quat = fcn(R)
Rot = zeros(3,3);
Rot = [R(1), R(2), R(3); R(4), R(5), R(6); R(7), R(8), R(9); ];
quat = rotm2quat(Rot)';
